simulink model "VD_3x_PT30"  (R2018b)
settings: Solver=ode8  StartTime=0.0  StopTime=0.7  RelTol=1e-3
undefined symbols (not defined in the file): C, L, R
libraries: powerlib x12, powerlib_meascontrol x6, peRmsMeasurement x2
settings Model: Creator=Anton  LastModifiedBy=VID Company
settings SFSimCC: SimUseLocalCustomCode=off
settings RTWCC: RTWUseLocalCustomCode=off
settings CodeAppCC: StateflowObjectComments=on
settings SimscapeCC: SimscapeNormalizeSystem=off

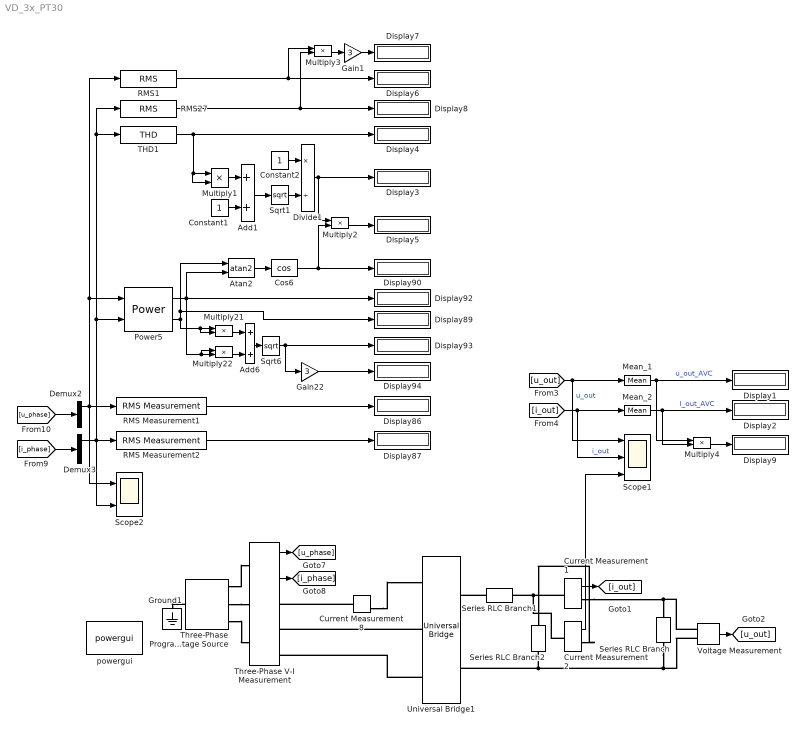
== system VD_3x_PT30 ==
  Add1 : Sum
  Add6 : Sum
  Atan2 : Trigonometry  Operator=atan2
  Constant1 : Constant
  Constant2 : Constant
  Cos6 : Trigonometry  Operator=cos
  Current Measurement1 : powerlib/Measurements/Current Measurement  PhasorSimulation=off  OutputType=Complex  PSBequivalent=0
  Current Measurement2 : powerlib/Measurements/Current Measurement  PhasorSimulation=off  OutputType=Complex  PSBequivalent=0
  Current Measurement8 : powerlib/Measurements/Current Measurement  PhasorSimulation=off  OutputType=Complex  PSBequivalent=0
  Demux2 : Demux  Outputs=3
  Demux3 : Demux  Outputs=3
  Display{1..9,86..87,89..90,92..94} (16 alike) : Display
  Divide1 : Product  Inputs=*/
  Gain1 : Gain  Gain=3
  Gain22 : Gain  Gain=3
  Ground1 : powerlib/Elements/Ground  LConnTagsString=a
  Mean_1 : powerlib_meascontrol/Measurements/Mean  Freq=300  Vinit=0  Ts=0
  Mean_2 : powerlib_meascontrol/Measurements/Mean  Freq=300  Vinit=0  Ts=0
  Multiply{1..4,21..22} (6 alike) : Product
  Power5 : powerlib_meascontrol/Measurements/Power  Freq=50  Vinit=[1, 0]  Iinit=[1, 0]  Ts=0
      settings: SourceProductName=Simscape Power Systems
  RMS Measurement1 : peRmsMeasurement/RMS Measurement  LabelModeActiveChoice=Harmonic  F=50  SpecifyHarmonics=on  K=[1]  Ts=0
  RMS Measurement2 : peRmsMeasurement/RMS Measurement  LabelModeActiveChoice=Harmonic  F=50  SpecifyHarmonics=on  K=[1]  Ts=0
  RMS1 : powerlib_meascontrol/Measurements/RMS  TrueRMS=on  Freq=50  RMSInit=0  Ts=0
  RMS27 : powerlib_meascontrol/Measurements/RMS  TrueRMS=on  Freq=50  RMSInit=0  Ts=0
  Scope1 : Scope  NumInputPorts=3
  Scope2 : Scope  NumInputPorts=2
  Series RLC Branch : powerlib/Elements/Series RLC Branch  LConnTagsString=__new0  RConnTagsString=__new0  BranchType=R  Resistance=R  Inductance=250e-6  SetiL0=off  InitialCurrent=0  Capacitance=1e-6  Setx0=off  InitialVoltage=0  Measurements=None
  Series RLC Branch1 : powerlib/Elements/Series RLC Branch  LConnTagsString=__new0  RConnTagsString=__new0  BranchType=L  Resistance=10  Inductance=L  SetiL0=off  InitialCurrent=0  Capacitance=1e-6  Setx0=off  InitialVoltage=0  Measurements=None
  Series RLC Branch2 : powerlib/Elements/Series RLC Branch  LConnTagsString=__new0  RConnTagsString=__new0  BranchType=RC  Resistance=10e-3  Inductance=250e-6  SetiL0=off  InitialCurrent=0  Capacitance=C  Setx0=on  InitialVoltage=U  Measurements=None
  Sqrt1 : Sqrt  SaturateOnIntegerOverflow=on
  Sqrt6 : Sqrt  SaturateOnIntegerOverflow=on
  THD1 : powerlib_meascontrol/Measurements/THD  Freq=50  Ts=0
  Three-Phase Programmable Voltage Source : powerlib/Electrical Sources/Three-Phase Programmable Voltage Source  PositiveSequence=[670 0 50]  VariationEntity=None  VariationType=Table of time-amplitude pairs  VariationTypeAlt=Step  VariationStep=0.5  VariationRate=10  VariationMagnitude=0.3  VariationFrequency=2  VariationTiming=[1 2]  VariationPhaseA=off  Amplitudes=[1 0.8 1.2 1.0]  TimeValues=[0 0.1 0.15 0.2]  HarmonicGeneration=off  HarmonicA=[3 0.2 -25 0]  HarmonicB=[2 0.15 35 2]  Timing="[0.05  3]"  BusType=swing  Pref=0  Qref=0  Qmin=-inf  Qmax=inf
  Three-Phase V-I Measurement : powerlib/Measurements/Three-Phase V-I Measurement  VoltageMeasurement=phase-to-ground  SetLabelV=off  LabelV=Vabc  Vpu=off  VpuLL=off  CurrentMeasurement=yes  SetLabelI=off  LabelI=Iabc  Ipu=off  Pbase=100e6  Vbase=500e3  OutputType=Complex  PhasorSimulation=off  PSBequivalent=0
  Universal Bridge1 : powerlib/Power Electronics/Universal Bridge  Arms=3  SnubberResistance=1e5  SnubberCapacitance=inf  Device=Diodes  Ron=30e-3  Lon=0  ForwardVoltages="[  0  0  ]"  ForwardVoltage=1  GTOparameters=[ 10e-6 , 20e-6 ]  IGBTparameters=[ 1e-6 , 2e-6 ]  Measurements=None  Measurements_2=None  converterType=Rectifier
  Voltage Measurement : powerlib/Measurements/Voltage Measurement  PhasorSimulation=off  OutputType=Complex  PSBequivalent=0
  powergui : powerlib/powergui  Priority=1  SimulationMode=Discrete  SampleTime=1e-6  frequency=60  Iterations=50  frequencyindice=0  Pbase=100e6  ErrMax=1e-4  UnitsV=kV  UnitsW=MW  buscounter=0  FunctionMessages=off  echomessages=off  EnableUseOfTLC=off  CurrentSourceSwitches=off  DisableSnubberDevices=off  DisableRonSwitches=off  DisableVfSwitches=off  DisplayEquations=off  SolverType=Tustin/Backward Euler (TBE)  Interpol=off  ExternalGateDelay=off  methode=off  Ts=100  x0status=blocks  SPID=off  SwTol=0  HookPort=off  RestoreLinks=warning  ResistiveCurrentMeasurement=off  Frange=[0:2:500]  Ylog=off  Xlog=on  ShowGrid=off  save=off  variable=ZData  structure=logsout  ZoomFFT=on  StartTime=0.67  cycles=5  DisplayStyle=1  fundamental=300  FreqAxis=off  MaxFrequency=1000  frequencyindicesteady=1  RmsSteady=1  display=off
  wires:
  Three-Phase V-I Measurement/2 -> [i_phase]
  Three-Phase V-I Measurement/1 -> [u_phase]
  [i_phase] -> Demux3/1
  Gain22/1 -> Display94/1
  Sqrt6/1 -> Display93/1, Gain22/1
  Demux2/1 -> Scope2/1, RMS Measurement1/1, RMS1/1, Power5/1
  Add6/1 -> Sqrt6/1
  Atan2/1 -> Cos6/1
  Power5/2 -> Atan2/1, Display89/1, Multiply21/2, Multiply21/1
  Demux3/1 -> Scope2/2, RMS Measurement2/1, THD1/1, RMS27/1, Power5/2
  Multiply21/1 -> Add6/1
  Cos6/1 -> Multiply2/2, Display90/1
  [u_phase] -> Demux2/1
  Multiply22/1 -> Add6/2
  RMS Measurement1/1 -> Display86/1
  RMS Measurement2/1 -> Display87/1
  Power5/1 -> Atan2/2, Multiply22/1, Multiply22/2, Display92/1
  Voltage Measurement/1 -> [u_out]
  [i_out] -> Mean_2/1, Scope1/2  "i_out"
  [u_out] -> Mean_1/1, Scope1/1  "u_out"
  Multiply1/1 -> Add1/1
  Constant2/1 -> Divide1/1
  Add1/1 -> Sqrt1/1
  Sqrt1/1 -> Divide1/2
  Divide1/1 -> Multiply2/1, Display3/1
  Constant1/1 -> Add1/2
  THD1/1 -> Multiply1/2, Multiply1/1, Display4/1
  RMS27/1 -> Multiply3/2, Display8/1
  Multiply2/1 -> Display5/1
  RMS1/1 -> Multiply3/1, Display6/1
  Gain1/1 -> Display7/1
  Multiply3/1 -> Gain1/1
  Mean_1/1 -> Display1/1, Multiply4/1  "u_out_AVC"
  Mean_2/1 -> Display2/1, Multiply4/2  "I_out_AVC"
  Multiply4/1 -> Display9/1
  Current Measurement1/1 -> [i_out]
  Current Measurement2/1 -> Scope1/3
  connections:
  Current Measurement8/LConn1 -- Three-Phase V-I Measurement/RConn1
  Universal Bridge1/LConn3 -- Three-Phase V-I Measurement/RConn3
  Universal Bridge1/LConn2 -- Three-Phase V-I Measurement/RConn2
  Three-Phase Programmable Voltage Source/RConn1 -- Three-Phase V-I Measurement/LConn1
  Three-Phase Programmable Voltage Source/LConn1 -- Ground1/LConn1
  Current Measurement8/RConn1 -- Universal Bridge1/LConn1
  Three-Phase Programmable Voltage Source/RConn3 -- Three-Phase V-I Measurement/LConn3
  Three-Phase Programmable Voltage Source/RConn2 -- Three-Phase V-I Measurement/LConn2
  Series RLC Branch/RConn1 -- Universal Bridge1/RConn2 -- Series RLC Branch2/RConn1 -- Voltage Measurement/LConn2
  Voltage Measurement/LConn1 -- Current Measurement1/RConn1 -- Series RLC Branch/LConn1
  Series RLC Branch1/LConn1 -- Universal Bridge1/RConn1
  Current Measurement1/LConn1 -- Current Measurement2/LConn1 -- Series RLC Branch1/RConn1
  Current Measurement2/RConn1 -- Series RLC Branch2/LConn1
